simulink model "HVPS230PFC"  (R2022b)
settings: configuration reference "ModelConfig_var" (kept outside this file)
undefined symbols (not defined in the file): InputCircuit
libraries: FMIKit_blocks x1
settings Model: Creator=KIRTACA  LastModifiedBy=BEDNASA
settings ConfigSetRef: SourceName=ModelConfig_var  SourceLocation=Base Workspace

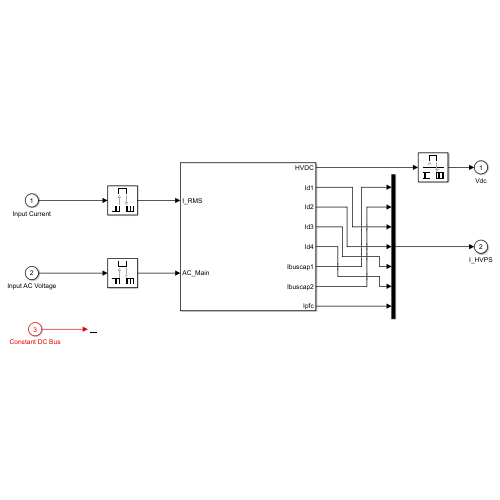
[thumbnail: Simulink's stored preview of the top-level diagram]
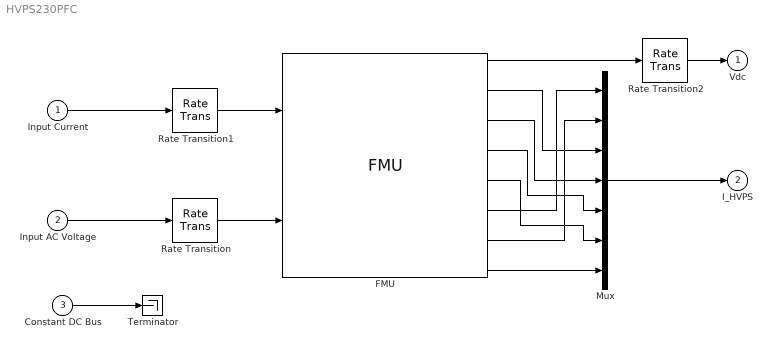
== system HVPS230PFC ==
  Input Current : Inport
  Input AC Voltage : Inport  Port=2
  Constant DC Bus : Inport  Port=3
  FMU : FMIKit_blocks/FMU
  Mux : Mux  Inputs=7
  Rate Transition : RateTransition  InitialCondition=InputCircuit.Vr  OutPortSampleTime=TimeSteps.InputCircuitStep
  Rate Transition1 : RateTransition  OutPortSampleTime=TimeSteps.InputCircuitStep
  Rate Transition2 : RateTransition  InitialCondition=InputCircuit.Vdc_i  OutPortSampleTime=TimeSteps.ModelStep
  Terminator : Terminator
  Vdc : Outport  VectorParamsAs1DForOutWhenUnconnected=off
  I_HVPS : Outport  Port=2  VectorParamsAs1DForOutWhenUnconnected=off
  wires:
  Input AC Voltage/1 -> Rate Transition/1
  Input Current/1 -> Rate Transition1/1
  Rate Transition2/1 -> Vdc/1
  Constant DC Bus/1 -> Terminator/1
  Rate Transition1/1 -> FMU/1
  Rate Transition/1 -> FMU/2
  FMU/1 -> Rate Transition2/1
  FMU/5 -> Mux/6
  FMU/2 -> Mux/3
  FMU/7 -> Mux/2
  FMU/3 -> Mux/4
  Mux/1 -> I_HVPS/1
  FMU/4 -> Mux/5
  FMU/8 -> Mux/7
  FMU/6 -> Mux/1
